simulink subsystem "getAccelData"  (R2024a)
settings: Solver=VariableStepAuto  StartTime=0.0  StopTime=10.0  RelTol=1e-3
undefined symbols (not defined in the file or in its folder): bits
libraries: stm32blockslib x8
settings Model: Creator=Peter  LastModifiedBy=Peter

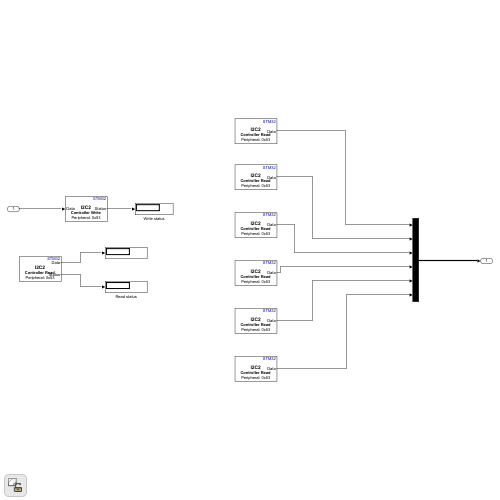
[thumbnail: Simulink's stored preview of the top-level diagram]
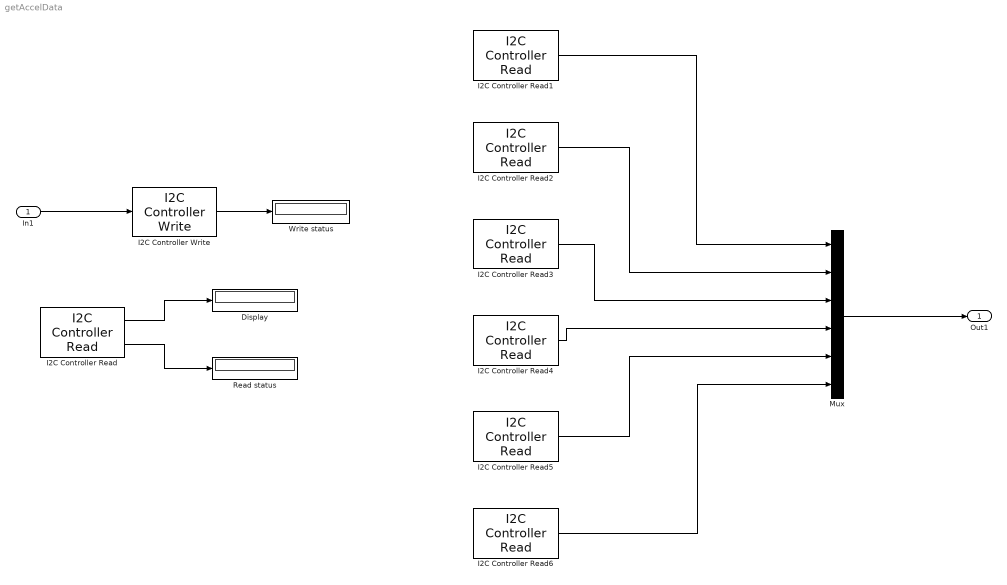
== system getAccelData ==
  In1 : Inport
  Display : Display
      settings: Format=hex (Stored Integer)
  I2C Controller Read : stm32blockslib/I2C Controller Read  I2CModule=I2C2  Mode=Controller  AddressingMode=7-bits  PeripheralByteOrder=LittleEndian  OwnPeripheralAddress=uint8(170)  PeripheralAddressVia=Dialog  PeripheralAddress=hex2dec('53')  RegisterAddressMode=on  RegisterAddressVia=Dialog  RegisterAddress=uint8(hex2dec('2D'))  RepeatedStart=off  NoAck=off  OutputStatus=on  BlockMode=Receive  DataType=uint8  DataLength=1  Timeout=0.001  SampleTime=0.1
      settings: LibrarySourceBlock=stm32f7xxblockslib/I2C Controller Read
  I2C Controller Read1 : stm32blockslib/I2C Controller Read  I2CModule=I2C2  Mode=Controller  AddressingMode=7-bits  PeripheralByteOrder=LittleEndian  OwnPeripheralAddress=uint8(170)  PeripheralAddressVia=Dialog  PeripheralAddress=hex2dec('53')  RegisterAddressMode=on  RegisterAddressVia=Dialog  RegisterAddress=uint8(hex2dec('32'))  RepeatedStart=off  NoAck=off  OutputStatus=off  BlockMode=Receive  DataType=uint8  DataLength=1  Timeout=0.001  SampleTime=inf
      settings: LibrarySourceBlock=stm32f7xxblockslib/I2C Controller Read
  I2C Controller Read2 : stm32blockslib/I2C Controller Read  I2CModule=I2C2  Mode=Controller  AddressingMode=7-bits  PeripheralByteOrder=LittleEndian  OwnPeripheralAddress=uint8(170)  PeripheralAddressVia=Dialog  PeripheralAddress=hex2dec('53')  RegisterAddressMode=on  RegisterAddressVia=Dialog  RegisterAddress=uint8(hex2dec('33'))  RepeatedStart=off  NoAck=off  OutputStatus=off  BlockMode=Receive  DataType=uint8  DataLength=1  Timeout=0.001  SampleTime=inf
      settings: LibrarySourceBlock=stm32f7xxblockslib/I2C Controller Read
  I2C Controller Read3 : stm32blockslib/I2C Controller Read  I2CModule=I2C2  Mode=Controller  AddressingMode=7-bits  PeripheralByteOrder=LittleEndian  OwnPeripheralAddress=uint8(170)  PeripheralAddressVia=Dialog  PeripheralAddress=hex2dec('53')  RegisterAddressMode=on  RegisterAddressVia=Dialog  RegisterAddress=uint8(hex2dec('34'))  RepeatedStart=off  NoAck=off  OutputStatus=off  BlockMode=Receive  DataType=uint8  DataLength=1  Timeout=0.001  SampleTime=inf
      settings: LibrarySourceBlock=stm32f7xxblockslib/I2C Controller Read
  I2C Controller Read4 : stm32blockslib/I2C Controller Read  I2CModule=I2C2  Mode=Controller  AddressingMode=7-bits  PeripheralByteOrder=LittleEndian  OwnPeripheralAddress=uint8(170)  PeripheralAddressVia=Dialog  PeripheralAddress=hex2dec('53')  RegisterAddressMode=on  RegisterAddressVia=Dialog  RegisterAddress=uint8(hex2dec('35'))  RepeatedStart=off  NoAck=off  OutputStatus=off  BlockMode=Receive  DataType=uint8  DataLength=1  Timeout=0.001  SampleTime=inf
      settings: LibrarySourceBlock=stm32f7xxblockslib/I2C Controller Read
  I2C Controller Read5 : stm32blockslib/I2C Controller Read  I2CModule=I2C2  Mode=Controller  AddressingMode=7-bits  PeripheralByteOrder=LittleEndian  OwnPeripheralAddress=uint8(170)  PeripheralAddressVia=Dialog  PeripheralAddress=hex2dec('53')  RegisterAddressMode=on  RegisterAddressVia=Dialog  RegisterAddress=uint8(hex2dec('36'))  RepeatedStart=off  NoAck=off  OutputStatus=off  BlockMode=Receive  DataType=uint8  DataLength=1  Timeout=0.001  SampleTime=inf
      settings: LibrarySourceBlock=stm32f7xxblockslib/I2C Controller Read
  I2C Controller Read6 : stm32blockslib/I2C Controller Read  I2CModule=I2C2  Mode=Controller  AddressingMode=7-bits  PeripheralByteOrder=LittleEndian  OwnPeripheralAddress=uint8(170)  PeripheralAddressVia=Dialog  PeripheralAddress=hex2dec('53')  RegisterAddressMode=on  RegisterAddressVia=Dialog  RegisterAddress=uint8(hex2dec('37'))  RepeatedStart=off  NoAck=off  OutputStatus=off  BlockMode=Receive  DataType=uint8  DataLength=1  Timeout=0.001  SampleTime=inf
      settings: LibrarySourceBlock=stm32f7xxblockslib/I2C Controller Read
  I2C Controller Write : stm32blockslib/I2C Controller Write  I2CModule=I2C2  Mode=Controller  AddressingMode=7-bits  PeripheralByteOrder=LittleEndian  OwnPeripheralAddress=uint8(170)  PeripheralAddressVia=Dialog  PeripheralAddress=hex2dec('53')  RegisterAddressMode=on  RegisterAddressVia=Dialog  RegisterAddress=uint8(hex2dec('2D'))  RepeatedStart=off  NoAck=off  OutputStatus=on  BlockMode=Transmit  DataType=uint8  DataLength=1  Timeout=0.001  SampleTime=-1
      settings: LibrarySourceBlock=stm32f7xxblockslib/I2C Controller Write
  Mux : Mux  Inputs=6
  Read status : Display
      settings: Format=hex (Stored Integer)
  Write status : Display
      settings: Format=hex (Stored Integer)
  Out1 : Outport  VectorParamsAs1DForOutWhenUnconnected=off
  wires:
  I2C Controller Write/1 -> Write status/1
  I2C Controller Read/1 -> Display/1
  In1/1 -> I2C Controller Write/1
  I2C Controller Read1/1 -> Mux/1
  I2C Controller Read/2 -> Read status/1
  I2C Controller Read2/1 -> Mux/2
  I2C Controller Read4/1 -> Mux/4
  I2C Controller Read6/1 -> Mux/6
  I2C Controller Read5/1 -> Mux/5
  Mux/1 -> Out1/1
  I2C Controller Read3/1 -> Mux/3
